simulink model "snb_bc"  (R2012b)
settings: Solver=FixedStepDiscrete  SolverMode=SingleTasking  StartTime=0.0  StopTime=10000  RelTol=1e-3
undefined symbols (not defined in the file): Down, pfb_coeff_gen_calc, Up
libraries: xbsIndex_r4 x19640, casper_library_misc x44, casper_library_delays x18, casper_library_communications x8, xps_library x3
(part 79 of 163)

== system snb_bc/pfb_fft/pfb_fir_generic/pfb_fir_taps/delay_bram ==
  addr : Inport
  din : Inport  Port=2
  we : Inport  Port=3
  en : Inport  Port=4
  bram{0..125} (126 alike) : xbsIndex_r4/Single Port RAM  depth=8192  initVector=getfield(get_param(gcb, 'UserData'), 'initVector')  distributed_mem=Block RAM  write_mode=Read Before Write  rst=off  init_reg=0  en=on  latency=8  dbl_ovrd=off  optimize=Speed  block_type=spram
  ddin : xbsIndex_r4/Delay  rst=off  infoeditControl=Selection of Reset will increase slice count due to use of real FFs and instead of SRLs  en=off  latency=0  dbl_ovrd=off  reg_retiming=on  block_type=delay
  debus_addr : Subsystem  AncestorBlock=casper_library_flow_control/bus_expand  mask(bus_expand){mode=divisions of equal size, outputNum=126, outputWidth=[13 13 13 13 13 13 13 13 13 13 13 13 13 13 13 13 13 13 13 13 13 13 13 13 13 13 13 13 13 13 13 13 13 13 13 13 13 13 13 13 13 13 13 13 13 13 13 13 13 13 13 13 13 13 13 13 13 13 13 13 13 13 13 13 13 13 13 13 13 13 13 13 13 13 13 13 13 13 13 13 13 13 13 13 13 13 13 13 13 13 13 13 13 13 13 13 13 13 13 13 13 13 13 13 13 13 13 13 13 13 13 13 13 13 13 13 13 13 13 13 13 13 13 13 13 13], outputBinaryPt=[0 0 0 0 0 0 0 0 0 0 0 0 0 0 0 0 0 0 0 0 0 0 0 0 0 0 0 0 0 0 0 0 0 0 0 0 0 0 0 0 0 0 0 0 0 0 0 0 0 0 0 0 0 0 0 0 0 0 0 0 0 0 0 0 0 0 0 0 0 0 0 0 0 0 0 0 0 0 0 0 0 0 0 0 0 0 0 0 0 0 0 0 0 0 0 0 0 0 0 0 0 0 0 0 0 0 0 0 0 0 0 0 0 0 0 0 0 0 0 0 0 0 0 0 0 0], outputArithmeticType=[0 0 0 0 0 0 0 0 0 0 0 0 0 0 0 0 0 0 0 0 0 0 0 0 0 0 0 0 0 0 0 0 0 0 0 0 0 0 0 0 0 0 0 0 0 0 0 0 0 0 0 0 0 0 0 0 0 0 0 0 0 0 0 0 0 0 0 0 0 0 0 0 0 0 0 0 0 0 0 0 0 0 0 0 0 0 0 0 0 0 0 0 0 0 0 0 0 0 0 0 0 0 0 0 0 0 0 0 0 0 0 0 0 0 0 0 0 0 0 0 0 0 0 0 0 0], show_format=on, outputToWorkspace=off, variablePrefix=, outputToModelAsWell=on}
      mask prompts: outputNum "Number of outputs:"; outputWidth "Output width:"; outputBinaryPt "Output binary point position:"; outputArithmeticType "Output arithmetic type (ufix=0, fix=1, bool=2):"; show_format "Print format string?"; outputToWorkspace "Output to workspace?"; variablePrefix "Variable name prefix:"; outputToModelAsWell "Output to model as well?"
      mask help:
      | Expands a 'bus' made using a bus_create or Xilinx
      | concat block.
      | The input will be divided into the specified number
      | of outputs with the specified arithmetic types.
      | Divisions are made from most significant bit.
      mask init: same as snb_bc/bus_expand10
      settings: AttributesFormatString=126 outputs: uf13.0,uf13.0,uf13.0,uf13.0,uf13.0,uf13.0,uf13.0,uf13.0,uf13.0,uf13.0,uf13.0,uf13.0,uf13.0,uf13.0,uf13.0,uf13.0,uf13.0,uf13.0,uf13.0,uf13.0,uf13.0,uf13.0,uf13.0,uf13.0,uf13.0,uf13.0,uf13.0,uf13.0,uf13.0,uf13.0,uf13.0,uf13.0,uf13.0,uf13.0,uf13.0,uf13.0,uf13.0,uf13.0,uf13.0,uf13.0,uf13.0,uf13.0,uf13.0,uf13.0,uf13.0,uf13.0,uf13.0,uf13.0,uf13.0,uf13.0,uf13.0,uf13.0,uf13.0,uf13.0,uf13.0,uf13.0,uf13.0,uf13.0,uf13.0,uf13.0,uf13.0,uf13.0,uf13.0,uf13.0,uf13.0,uf13.0,uf13.0,uf13.0,uf13.0,uf13.0,uf13.0,uf13.0,uf13.0,uf13.0,uf13.0,uf13.0,uf13.0,uf13.0,uf13.0,uf13.0,uf13.0,uf13.0,uf13.0,uf13.0,uf13.0,uf13.0,uf13.0,uf13.0,uf13.0,uf13.0,uf13.0,uf13.0,uf13.0,uf13.0,uf13.0,uf13.0,uf13.0,uf13.0,uf13.0,uf13.0,uf13.0,uf13.0,uf13.0,uf13.0,uf13.0,uf13.0,uf13.0,uf13.0,uf13.0,uf13.0,uf13.0,uf13.0,uf13.0,uf13.0,uf13.0,uf13.0,uf13.0,uf13.0,uf13.0,uf13.0,uf13.0,uf13.0,uf13.0,uf13.0,uf13.0,uf13.0,
      mask TypeOptions mode: divisions of equal size | divisions of arbitrary size
      mask Callback mode: bus_expand_callback();
      mask Callback outputWidth: bus_expand_callback();
      mask Callback outputToWorkspace: bus_expand_callback();
  debus_din : Subsystem  AncestorBlock=casper_library_flow_control/bus_expand  mask(bus_expand){mode=divisions of arbitrary size, outputNum=1, outputWidth=[4 4 4 4 4 4 4 4 4 4 4 4 4 4 4 4 4 4 4 4 4 4 4 4 4 4 4 4 4 4 4 4 4 4 4 4 4 4 4 4 4 4 4 4 4 4 4 4 4 4 4 4 4 4 4 4 4 4 4 4 4 4 4 4 4 4 4 4 4 4 4 4 4 4 4 4 4 4 4 4 4 4 4 4 4 4 4 4 4 4 4 4 4 4 4 4 4 4 4 4 4 4 4 4 4 4 4 4 4 4 4 4 4 4 4 4 4 4 4 4 4 4 4 4 4 4], outputBinaryPt=[0 0 0 0 0 0 0 0 0 0 0 0 0 0 0 0 0 0 0 0 0 0 0 0 0 0 0 0 0 0 0 0 0 0 0 0 0 0 0 0 0 0 0 0 0 0 0 0 0 0 0 0 0 0 0 0 0 0 0 0 0 0 0 0 0 0 0 0 0 0 0 0 0 0 0 0 0 0 0 0 0 0 0 0 0 0 0 0 0 0 0 0 0 0 0 0 0 0 0 0 0 0 0 0 0 0 0 0 0 0 0 0 0 0 0 0 0 0 0 0 0 0 0 0 0 0], outputArithmeticType=[0 0 0 0 0 0 0 0 0 0 0 0 0 0 0 0 0 0 0 0 0 0 0 0 0 0 0 0 0 0 0 0 0 0 0 0 0 0 0 0 0 0 0 0 0 0 0 0 0 0 0 0 0 0 0 0 0 0 0 0 0 0 0 0 0 0 0 0 0 0 0 0 0 0 0 0 0 0 0 0 0 0 0 0 0 0 0 0 0 0 0 0 0 0 0 0 0 0 0 0 0 0 0 0 0 0 0 0 0 0 0 0 0 0 0 0 0 0 0 0 0 0 0 0 0 0], show_format=on, outputToWorkspace=off, variablePrefix=, outputToModelAsWell=on}
      mask prompts: outputNum "Number of outputs:"; outputWidth "Output width [msb ... lsb]:"; outputBinaryPt "Output binary point position [msb ... lsb]:"; outputArithmeticType "Output arithmetic type (ufix=0, fix=1, bool=2) [msb ... lsb]:"; show_format "Print format string?"; outputToWorkspace "Output to workspace?"; variablePrefix "Variable name prefix:"; outputToModelAsWell "Output to model as well?"
      mask help:
      | Expands a 'bus' made using a bus_create or Xilinx
      | concat block.
      | The input will be divided into the specified number
      | of outputs with the specified arithmetic types.
      | Divisions are made from most significant bit.
      mask init: same as snb_bc/bus_expand10
      settings: AttributesFormatString=126 outputs: uf4.0,uf4.0,uf4.0,uf4.0,uf4.0,uf4.0,uf4.0,uf4.0,uf4.0,uf4.0,uf4.0,uf4.0,uf4.0,uf4.0,uf4.0,uf4.0,uf4.0,uf4.0,uf4.0,uf4.0,uf4.0,uf4.0,uf4.0,uf4.0,uf4.0,uf4.0,uf4.0,uf4.0,uf4.0,uf4.0,uf4.0,uf4.0,uf4.0,uf4.0,uf4.0,uf4.0,uf4.0,uf4.0,uf4.0,uf4.0,uf4.0,uf4.0,uf4.0,uf4.0,uf4.0,uf4.0,uf4.0,uf4.0,uf4.0,uf4.0,uf4.0,uf4.0,uf4.0,uf4.0,uf4.0,uf4.0,uf4.0,uf4.0,uf4.0,uf4.0,uf4.0,uf4.0,uf4.0,uf4.0,uf4.0,uf4.0,uf4.0,uf4.0,uf4.0,uf4.0,uf4.0,uf4.0,uf4.0,uf4.0,uf4.0,uf4.0,uf4.0,uf4.0,uf4.0,uf4.0,uf4.0,uf4.0,uf4.0,uf4.0,uf4.0,uf4.0,uf4.0,uf4.0,uf4.0,uf4.0,uf4.0,uf4.0,uf4.0,uf4.0,uf4.0,uf4.0,uf4.0,uf4.0,uf4.0,uf4.0,uf4.0,uf4.0,uf4.0,uf4.0,uf4.0,uf4.0,uf4.0,uf4.0,uf4.0,uf4.0,uf4.0,uf4.0,uf4.0,uf4.0,uf4.0,uf4.0,uf4.0,uf4.0,uf4.0,uf4.0,uf4.0,uf4.0,uf4.0,uf4.0,uf4.0,uf4.0,
      mask TypeOptions mode: divisions of equal size | divisions of arbitrary size
      mask Callback mode: bus_expand_callback();
      mask Callback outputWidth: bus_expand_callback();
      mask Callback outputToWorkspace: bus_expand_callback();
  debus_en : Subsystem  AncestorBlock=casper_library_flow_control/bus_expand  mask(bus_expand){mode=divisions of equal size, outputNum=126, outputWidth=[1 1 1 1 1 1 1 1 1 1 1 1 1 1 1 1 1 1 1 1 1 1 1 1 1 1 1 1 1 1 1 1 1 1 1 1 1 1 1 1 1 1 1 1 1 1 1 1 1 1 1 1 1 1 1 1 1 1 1 1 1 1 1 1 1 1 1 1 1 1 1 1 1 1 1 1 1 1 1 1 1 1 1 1 1 1 1 1 1 1 1 1 1 1 1 1 1 1 1 1 1 1 1 1 1 1 1 1 1 1 1 1 1 1 1 1 1 1 1 1 1 1 1 1 1 1], outputBinaryPt=[0 0 0 0 0 0 0 0 0 0 0 0 0 0 0 0 0 0 0 0 0 0 0 0 0 0 0 0 0 0 0 0 0 0 0 0 0 0 0 0 0 0 0 0 0 0 0 0 0 0 0 0 0 0 0 0 0 0 0 0 0 0 0 0 0 0 0 0 0 0 0 0 0 0 0 0 0 0 0 0 0 0 0 0 0 0 0 0 0 0 0 0 0 0 0 0 0 0 0 0 0 0 0 0 0 0 0 0 0 0 0 0 0 0 0 0 0 0 0 0 0 0 0 0 0 0], outputArithmeticType=[2 2 2 2 2 2 2 2 2 2 2 2 2 2 2 2 2 2 2 2 2 2 2 2 2 2 2 2 2 2 2 2 2 2 2 2 2 2 2 2 2 2 2 2 2 2 2 2 2 2 2 2 2 2 2 2 2 2 2 2 2 2 2 2 2 2 2 2 2 2 2 2 2 2 2 2 2 2 2 2 2 2 2 2 2 2 2 2 2 2 2 2 2 2 2 2 2 2 2 2 2 2 2 2 2 2 2 2 2 2 2 2 2 2 2 2 2 2 2 2 2 2 2 2 2 2], show_format=on, outputToWorkspace=off, variablePrefix=, outputToModelAsWell=on}
      mask prompts: outputNum "Number of outputs:"; outputWidth "Output width:"; outputBinaryPt "Output binary point position:"; outputArithmeticType "Output arithmetic type (ufix=0, fix=1, bool=2):"; show_format "Print format string?"; outputToWorkspace "Output to workspace?"; variablePrefix "Variable name prefix:"; outputToModelAsWell "Output to model as well?"
      mask help:
      | Expands a 'bus' made using a bus_create or Xilinx
      | concat block.
      | The input will be divided into the specified number
      | of outputs with the specified arithmetic types.
      | Divisions are made from most significant bit.
      mask init: same as snb_bc/bus_expand10
      settings: AttributesFormatString=126 outputs: b,b,b,b,b,b,b,b,b,b,b,b,b,b,b,b,b,b,b,b,b,b,b,b,b,b,b,b,b,b,b,b,b,b,b,b,b,b,b,b,b,b,b,b,b,b,b,b,b,b,b,b,b,b,b,b,b,b,b,b,b,b,b,b,b,b,b,b,b,b,b,b,b,b,b,b,b,b,b,b,b,b,b,b,b,b,b,b,b,b,b,b,b,b,b,b,b,b,b,b,b,b,b,b,b,b,b,b,b,b,b,b,b,b,b,b,b,b,b,b,b,b,b,b,b,b,
      mask TypeOptions mode: divisions of equal size | divisions of arbitrary size
      mask Callback mode: bus_expand_callback();
      mask Callback outputWidth: bus_expand_callback();
      mask Callback outputToWorkspace: bus_expand_callback();
  debus_we : Subsystem  AncestorBlock=casper_library_flow_control/bus_expand  mask(bus_expand){mode=divisions of equal size, outputNum=126, outputWidth=[1 1 1 1 1 1 1 1 1 1 1 1 1 1 1 1 1 1 1 1 1 1 1 1 1 1 1 1 1 1 1 1 1 1 1 1 1 1 1 1 1 1 1 1 1 1 1 1 1 1 1 1 1 1 1 1 1 1 1 1 1 1 1 1 1 1 1 1 1 1 1 1 1 1 1 1 1 1 1 1 1 1 1 1 1 1 1 1 1 1 1 1 1 1 1 1 1 1 1 1 1 1 1 1 1 1 1 1 1 1 1 1 1 1 1 1 1 1 1 1 1 1 1 1 1 1], outputBinaryPt=[0 0 0 0 0 0 0 0 0 0 0 0 0 0 0 0 0 0 0 0 0 0 0 0 0 0 0 0 0 0 0 0 0 0 0 0 0 0 0 0 0 0 0 0 0 0 0 0 0 0 0 0 0 0 0 0 0 0 0 0 0 0 0 0 0 0 0 0 0 0 0 0 0 0 0 0 0 0 0 0 0 0 0 0 0 0 0 0 0 0 0 0 0 0 0 0 0 0 0 0 0 0 0 0 0 0 0 0 0 0 0 0 0 0 0 0 0 0 0 0 0 0 0 0 0 0], outputArithmeticType=[2 2 2 2 2 2 2 2 2 2 2 2 2 2 2 2 2 2 2 2 2 2 2 2 2 2 2 2 2 2 2 2 2 2 2 2 2 2 2 2 2 2 2 2 2 2 2 2 2 2 2 2 2 2 2 2 2 2 2 2 2 2 2 2 2 2 2 2 2 2 2 2 2 2 2 2 2 2 2 2 2 2 2 2 2 2 2 2 2 2 2 2 2 2 2 2 2 2 2 2 2 2 2 2 2 2 2 2 2 2 2 2 2 2 2 2 2 2 2 2 2 2 2 2 2 2], show_format=on, outputToWorkspace=off, variablePrefix=, outputToModelAsWell=on}
      mask prompts: outputNum "Number of outputs:"; outputWidth "Output width:"; outputBinaryPt "Output binary point position:"; outputArithmeticType "Output arithmetic type (ufix=0, fix=1, bool=2):"; show_format "Print format string?"; outputToWorkspace "Output to workspace?"; variablePrefix "Variable name prefix:"; outputToModelAsWell "Output to model as well?"
      mask help:
      | Expands a 'bus' made using a bus_create or Xilinx
      | concat block.
      | The input will be divided into the specified number
      | of outputs with the specified arithmetic types.
      | Divisions are made from most significant bit.
      mask init: same as snb_bc/bus_expand10
      settings: AttributesFormatString=126 outputs: b,b,b,b,b,b,b,b,b,b,b,b,b,b,b,b,b,b,b,b,b,b,b,b,b,b,b,b,b,b,b,b,b,b,b,b,b,b,b,b,b,b,b,b,b,b,b,b,b,b,b,b,b,b,b,b,b,b,b,b,b,b,b,b,b,b,b,b,b,b,b,b,b,b,b,b,b,b,b,b,b,b,b,b,b,b,b,b,b,b,b,b,b,b,b,b,b,b,b,b,b,b,b,b,b,b,b,b,b,b,b,b,b,b,b,b,b,b,b,b,b,b,b,b,b,b,
      mask TypeOptions mode: divisions of equal size | divisions of arbitrary size
      mask Callback mode: bus_expand_callback();
      mask Callback outputWidth: bus_expand_callback();
      mask Callback outputToWorkspace: bus_expand_callback();
  den : xbsIndex_r4/Delay  rst=off  infoeditControl=Selection of Reset will increase slice count due to use of real FFs and instead of SRLs  en=off  latency=8  dbl_ovrd=off  reg_retiming=on  block_type=delay
  din_bussify : Subsystem  AncestorBlock=casper_library_flow_control/bus_create  mask(bus_create){inputNum=126}
      mask prompts: inputNum "Number of inputs:"
      mask init:
      | bus_create_init(gcb,...
      |     'inputNum', inputNum);
  rep_addr : Subsystem  AncestorBlock=casper_library_bus/bus_replicate  mask(bus_replicate){replication=126, latency=9, misc=off, implementation=core}
      mask prompts: replication "replication factor"; misc "misc support"; implementation "delay implementation"
      mask help: Output bus formed by replicating input bus a number of times
      mask init:
      | bus_replicate_init(gcb, ...
      |     'replication', replication, ...
      |     'latency', latency, ...
      |     'implementation', implementation, ...
      |     'misc', misc);
      mask TypeOptions implementation: core | behavioral
  rep_en : Subsystem  AncestorBlock=casper_library_bus/bus_replicate  mask(bus_replicate){replication=126, latency=9, misc=off, implementation=core}
      mask prompts: replication "replication factor"; misc "misc support"; implementation "delay implementation"
      mask help: Output bus formed by replicating input bus a number of times
      mask init:
      | bus_replicate_init(gcb, ...
      |     'replication', replication, ...
      |     'latency', latency, ...
      |     'implementation', implementation, ...
      |     'misc', misc);
      mask TypeOptions implementation: core | behavioral
  rep_we : Subsystem  AncestorBlock=casper_library_bus/bus_replicate  mask(bus_replicate){replication=126, latency=0, misc=off, implementation=behavioral}
      mask prompts: replication "replication factor"; misc "misc support"; implementation "delay implementation"
      mask help: Output bus formed by replicating input bus a number of times
      mask init:
      | bus_replicate_init(gcb, ...
      |     'replication', replication, ...
      |     'latency', latency, ...
      |     'implementation', implementation, ...
      |     'misc', misc);
      mask TypeOptions implementation: core | behavioral
  dout : Outport
  dvalid : Outport  Port=2
  wires:
  addr/1 -> rep_addr/1(in)
  din/1 -> ddin/1
  we/1 -> rep_we/1(in)
  en/1 -> rep_en/1(in)
  rep_addr/1(out) -> debus_addr/1(bus_in)
  ddin/1 -> debus_din/1(bus_in)
  rep_we/1(out) -> debus_we/1(bus_in)
  rep_en/1(out) -> debus_en/1(bus_in)
  debus_addr/1(msb_out126) -> bram0/1
  debus_din/1(msb_out126) -> bram0/2
  debus_we/1(msb_out126) -> bram0/3
  debus_en/1(msb_out126) -> bram0/4
  debus_addr/2(out125) -> bram1/1
  debus_din/2(out125) -> bram1/2
  debus_we/2(out125) -> bram1/3
  debus_en/2(out125) -> bram1/4
  debus_addr/3(out124) -> bram2/1
  debus_din/3(out124) -> bram2/2
  debus_we/3(out124) -> bram2/3
  debus_en/3(out124) -> bram2/4
  debus_addr/4(out123) -> bram3/1
  debus_din/4(out123) -> bram3/2
  debus_we/4(out123) -> bram3/3
  debus_en/4(out123) -> bram3/4
  debus_addr/5(out122) -> bram4/1
  debus_din/5(out122) -> bram4/2
  debus_we/5(out122) -> bram4/3
  debus_en/5(out122) -> bram4/4
  debus_addr/6(out121) -> bram5/1
  debus_din/6(out121) -> bram5/2
  debus_we/6(out121) -> bram5/3
  debus_en/6(out121) -> bram5/4
  debus_addr/7(out120) -> bram6/1
  debus_din/7(out120) -> bram6/2
  debus_we/7(out120) -> bram6/3
  debus_en/7(out120) -> bram6/4
  debus_addr/8(out119) -> bram7/1
  debus_din/8(out119) -> bram7/2
  debus_we/8(out119) -> bram7/3
  debus_en/8(out119) -> bram7/4
  debus_addr/9(out118) -> bram8/1
  debus_din/9(out118) -> bram8/2
  debus_we/9(out118) -> bram8/3
  debus_en/9(out118) -> bram8/4
  debus_addr/10(out117) -> bram9/1
  debus_din/10(out117) -> bram9/2
  debus_we/10(out117) -> bram9/3
  debus_en/10(out117) -> bram9/4
  debus_addr/11(out116) -> bram10/1
  debus_din/11(out116) -> bram10/2
  debus_we/11(out116) -> bram10/3
  debus_en/11(out116) -> bram10/4
  debus_addr/12(out115) -> bram11/1
  debus_din/12(out115) -> bram11/2
  debus_we/12(out115) -> bram11/3
  debus_en/12(out115) -> bram11/4
  debus_addr/13(out114) -> bram12/1
  debus_din/13(out114) -> bram12/2
  debus_we/13(out114) -> bram12/3
  debus_en/13(out114) -> bram12/4
  debus_addr/14(out113) -> bram13/1
  debus_din/14(out113) -> bram13/2
  debus_we/14(out113) -> bram13/3
  debus_en/14(out113) -> bram13/4
  debus_addr/15(out112) -> bram14/1
  debus_din/15(out112) -> bram14/2
  debus_we/15(out112) -> bram14/3
  debus_en/15(out112) -> bram14/4
  debus_addr/16(out111) -> bram15/1
  debus_din/16(out111) -> bram15/2
  debus_we/16(out111) -> bram15/3
  debus_en/16(out111) -> bram15/4
  debus_addr/17(out110) -> bram16/1
  debus_din/17(out110) -> bram16/2
  debus_we/17(out110) -> bram16/3
  debus_en/17(out110) -> bram16/4
  debus_addr/18(out109) -> bram17/1
  debus_din/18(out109) -> bram17/2
  debus_we/18(out109) -> bram17/3
  debus_en/18(out109) -> bram17/4
  debus_addr/19(out108) -> bram18/1
  debus_din/19(out108) -> bram18/2
  debus_we/19(out108) -> bram18/3
  debus_en/19(out108) -> bram18/4
  debus_addr/20(out107) -> bram19/1
  debus_din/20(out107) -> bram19/2
  debus_we/20(out107) -> bram19/3
  debus_en/20(out107) -> bram19/4
  debus_addr/21(out106) -> bram20/1
  debus_din/21(out106) -> bram20/2
  debus_we/21(out106) -> bram20/3
  debus_en/21(out106) -> bram20/4
  debus_addr/22(out105) -> bram21/1
  debus_din/22(out105) -> bram21/2
  debus_we/22(out105) -> bram21/3
  debus_en/22(out105) -> bram21/4
  debus_addr/23(out104) -> bram22/1
  debus_din/23(out104) -> bram22/2
  debus_we/23(out104) -> bram22/3
  debus_en/23(out104) -> bram22/4
  debus_addr/24(out103) -> bram23/1
  debus_din/24(out103) -> bram23/2
  debus_we/24(out103) -> bram23/3
  debus_en/24(out103) -> bram23/4
  debus_addr/25(out102) -> bram24/1
  debus_din/25(out102) -> bram24/2
  debus_we/25(out102) -> bram24/3
  debus_en/25(out102) -> bram24/4
  debus_addr/26(out101) -> bram25/1
  debus_din/26(out101) -> bram25/2
  debus_we/26(out101) -> bram25/3
  debus_en/26(out101) -> bram25/4
  debus_addr/27(out100) -> bram26/1
  debus_din/27(out100) -> bram26/2
  debus_we/27(out100) -> bram26/3
  debus_en/27(out100) -> bram26/4
  debus_addr/28(out99) -> bram27/1
  debus_din/28(out99) -> bram27/2
  debus_we/28(out99) -> bram27/3
  debus_en/28(out99) -> bram27/4
  debus_addr/29(out98) -> bram28/1
  debus_din/29(out98) -> bram28/2
  debus_we/29(out98) -> bram28/3
  debus_en/29(out98) -> bram28/4
  debus_addr/30(out97) -> bram29/1
  debus_din/30(out97) -> bram29/2
  debus_we/30(out97) -> bram29/3
  debus_en/30(out97) -> bram29/4
  debus_addr/31(out96) -> bram30/1
  debus_din/31(out96) -> bram30/2
  debus_we/31(out96) -> bram30/3
  debus_en/31(out96) -> bram30/4
  debus_addr/32(out95) -> bram31/1
  debus_din/32(out95) -> bram31/2
  debus_we/32(out95) -> bram31/3
  debus_en/32(out95) -> bram31/4
  debus_addr/33(out94) -> bram32/1
  debus_din/33(out94) -> bram32/2
  debus_we/33(out94) -> bram32/3
  debus_en/33(out94) -> bram32/4
  debus_addr/34(out93) -> bram33/1
  debus_din/34(out93) -> bram33/2
  debus_we/34(out93) -> bram33/3
  debus_en/34(out93) -> bram33/4
  debus_addr/35(out92) -> bram34/1
  debus_din/35(out92) -> bram34/2
  debus_we/35(out92) -> bram34/3
  debus_en/35(out92) -> bram34/4
  debus_addr/36(out91) -> bram35/1
  debus_din/36(out91) -> bram35/2
  debus_we/36(out91) -> bram35/3
  debus_en/36(out91) -> bram35/4
  debus_addr/37(out90) -> bram36/1
  debus_din/37(out90) -> bram36/2
  debus_we/37(out90) -> bram36/3
  debus_en/37(out90) -> bram36/4
  debus_addr/38(out89) -> bram37/1
  debus_din/38(out89) -> bram37/2
  debus_we/38(out89) -> bram37/3
  debus_en/38(out89) -> bram37/4
  debus_addr/39(out88) -> bram38/1
  debus_din/39(out88) -> bram38/2
  debus_we/39(out88) -> bram38/3
  debus_en/39(out88) -> bram38/4
  debus_addr/40(out87) -> bram39/1
  debus_din/40(out87) -> bram39/2
  debus_we/40(out87) -> bram39/3
  debus_en/40(out87) -> bram39/4
  debus_addr/41(out86) -> bram40/1
  debus_din/41(out86) -> bram40/2
  debus_we/41(out86) -> bram40/3
  debus_en/41(out86) -> bram40/4
  debus_addr/42(out85) -> bram41/1
  debus_din/42(out85) -> bram41/2
  debus_we/42(out85) -> bram41/3
  debus_en/42(out85) -> bram41/4
  debus_addr/43(out84) -> bram42/1
  debus_din/43(out84) -> bram42/2
  debus_we/43(out84) -> bram42/3
  debus_en/43(out84) -> bram42/4
  debus_addr/44(out83) -> bram43/1
  debus_din/44(out83) -> bram43/2
  debus_we/44(out83) -> bram43/3
  debus_en/44(out83) -> bram43/4
  debus_addr/45(out82) -> bram44/1
  debus_din/45(out82) -> bram44/2
  debus_we/45(out82) -> bram44/3
  debus_en/45(out82) -> bram44/4
  debus_addr/46(out81) -> bram45/1
  debus_din/46(out81) -> bram45/2
  debus_we/46(out81) -> bram45/3
  debus_en/46(out81) -> bram45/4
  debus_addr/47(out80) -> bram46/1
  debus_din/47(out80) -> bram46/2
  debus_we/47(out80) -> bram46/3
  debus_en/47(out80) -> bram46/4
  debus_addr/48(out79) -> bram47/1
  debus_din/48(out79) -> bram47/2
  debus_we/48(out79) -> bram47/3
  debus_en/48(out79) -> bram47/4
  debus_addr/49(out78) -> bram48/1
  debus_din/49(out78) -> bram48/2
  debus_we/49(out78) -> bram48/3
  debus_en/49(out78) -> bram48/4
  debus_addr/50(out77) -> bram49/1
  debus_din/50(out77) -> bram49/2
  debus_we/50(out77) -> bram49/3
  debus_en/50(out77) -> bram49/4
  debus_addr/51(out76) -> bram50/1
  debus_din/51(out76) -> bram50/2
  debus_we/51(out76) -> bram50/3
  debus_en/51(out76) -> bram50/4
  debus_addr/52(out75) -> bram51/1
  debus_din/52(out75) -> bram51/2
  debus_we/52(out75) -> bram51/3
  debus_en/52(out75) -> bram51/4
  debus_addr/53(out74) -> bram52/1
  debus_din/53(out74) -> bram52/2
  debus_we/53(out74) -> bram52/3
  debus_en/53(out74) -> bram52/4
  debus_addr/54(out73) -> bram53/1
  debus_din/54(out73) -> bram53/2
  debus_we/54(out73) -> bram53/3
  debus_en/54(out73) -> bram53/4
  debus_addr/55(out72) -> bram54/1
  debus_din/55(out72) -> bram54/2
  debus_we/55(out72) -> bram54/3
  debus_en/55(out72) -> bram54/4
  debus_addr/56(out71) -> bram55/1
  debus_din/56(out71) -> bram55/2
  debus_we/56(out71) -> bram55/3
  debus_en/56(out71) -> bram55/4
  debus_addr/57(out70) -> bram56/1
  debus_din/57(out70) -> bram56/2
  debus_we/57(out70) -> bram56/3
  debus_en/57(out70) -> bram56/4
  debus_addr/58(out69) -> bram57/1
  debus_din/58(out69) -> bram57/2
  debus_we/58(out69) -> bram57/3
  debus_en/58(out69) -> bram57/4
  debus_addr/59(out68) -> bram58/1
  debus_din/59(out68) -> bram58/2
  debus_we/59(out68) -> bram58/3
  debus_en/59(out68) -> bram58/4
  debus_addr/60(out67) -> bram59/1
  debus_din/60(out67) -> bram59/2
  debus_we/60(out67) -> bram59/3
  debus_en/60(out67) -> bram59/4
  debus_addr/61(out66) -> bram60/1
  debus_din/61(out66) -> bram60/2
  debus_we/61(out66) -> bram60/3
  debus_en/61(out66) -> bram60/4
  debus_addr/62(out65) -> bram61/1
  debus_din/62(out65) -> bram61/2
  debus_we/62(out65) -> bram61/3
  debus_en/62(out65) -> bram61/4
  debus_addr/63(out64) -> bram62/1
  debus_din/63(out64) -> bram62/2
  debus_we/63(out64) -> bram62/3
  debus_en/63(out64) -> bram62/4
  debus_addr/64(out63) -> bram63/1
  debus_din/64(out63) -> bram63/2
  debus_we/64(out63) -> bram63/3
  debus_en/64(out63) -> bram63/4
  debus_addr/65(out62) -> bram64/1
  debus_din/65(out62) -> bram64/2
  debus_we/65(out62) -> bram64/3
  debus_en/65(out62) -> bram64/4
  debus_addr/66(out61) -> bram65/1
  debus_din/66(out61) -> bram65/2
  debus_we/66(out61) -> bram65/3
  debus_en/66(out61) -> bram65/4
  debus_addr/67(out60) -> bram66/1
  debus_din/67(out60) -> bram66/2
  debus_we/67(out60) -> bram66/3
  debus_en/67(out60) -> bram66/4
  debus_addr/68(out59) -> bram67/1
  debus_din/68(out59) -> bram67/2
  debus_we/68(out59) -> bram67/3
  debus_en/68(out59) -> bram67/4
  debus_addr/69(out58) -> bram68/1
  debus_din/69(out58) -> bram68/2
  debus_we/69(out58) -> bram68/3
  debus_en/69(out58) -> bram68/4
  debus_addr/70(out57) -> bram69/1
  debus_din/70(out57) -> bram69/2
  debus_we/70(out57) -> bram69/3
  debus_en/70(out57) -> bram69/4
  debus_addr/71(out56) -> bram70/1
  debus_din/71(out56) -> bram70/2
  debus_we/71(out56) -> bram70/3
  debus_en/71(out56) -> bram70/4
  debus_addr/72(out55) -> bram71/1
  debus_din/72(out55) -> bram71/2
  debus_we/72(out55) -> bram71/3
  debus_en/72(out55) -> bram71/4
  debus_addr/73(out54) -> bram72/1
  debus_din/73(out54) -> bram72/2
  debus_we/73(out54) -> bram72/3
  debus_en/73(out54) -> bram72/4
  debus_addr/74(out53) -> bram73/1
  debus_din/74(out53) -> bram73/2
  debus_we/74(out53) -> bram73/3
  debus_en/74(out53) -> bram73/4
  debus_addr/75(out52) -> bram74/1
  debus_din/75(out52) -> bram74/2
  debus_we/75(out52) -> bram74/3
  debus_en/75(out52) -> bram74/4
  debus_addr/76(out51) -> bram75/1
  debus_din/76(out51) -> bram75/2
  debus_we/76(out51) -> bram75/3
  debus_en/76(out51) -> bram75/4
  debus_addr/77(out50) -> bram76/1
  debus_din/77(out50) -> bram76/2
  debus_we/77(out50) -> bram76/3
  debus_en/77(out50) -> bram76/4
  debus_addr/78(out49) -> bram77/1
  debus_din/78(out49) -> bram77/2
  debus_we/78(out49) -> bram77/3
  debus_en/78(out49) -> bram77/4
  debus_addr/79(out48) -> bram78/1
  debus_din/79(out48) -> bram78/2
  debus_we/79(out48) -> bram78/3
  debus_en/79(out48) -> bram78/4
  debus_addr/80(out47) -> bram79/1
  debus_din/80(out47) -> bram79/2
  debus_we/80(out47) -> bram79/3
  debus_en/80(out47) -> bram79/4
  debus_addr/81(out46) -> bram80/1
  debus_din/81(out46) -> bram80/2
  debus_we/81(out46) -> bram80/3
  debus_en/81(out46) -> bram80/4
  debus_addr/82(out45) -> bram81/1
  debus_din/82(out45) -> bram81/2
  debus_we/82(out45) -> bram81/3
  debus_en/82(out45) -> bram81/4
  debus_addr/83(out44) -> bram82/1
  debus_din/83(out44) -> bram82/2
  debus_we/83(out44) -> bram82/3
  debus_en/83(out44) -> bram82/4
  debus_addr/84(out43) -> bram83/1
  debus_din/84(out43) -> bram83/2
  debus_we/84(out43) -> bram83/3
  debus_en/84(out43) -> bram83/4
  debus_addr/85(out42) -> bram84/1
  debus_din/85(out42) -> bram84/2
  debus_we/85(out42) -> bram84/3
  debus_en/85(out42) -> bram84/4
  debus_addr/86(out41) -> bram85/1
  debus_din/86(out41) -> bram85/2
  debus_we/86(out41) -> bram85/3
  debus_en/86(out41) -> bram85/4
  debus_addr/87(out40) -> bram86/1
  debus_din/87(out40) -> bram86/2
  debus_we/87(out40) -> bram86/3
  debus_en/87(out40) -> bram86/4
  debus_addr/88(out39) -> bram87/1
  debus_din/88(out39) -> bram87/2
  debus_we/88(out39) -> bram87/3
  debus_en/88(out39) -> bram87/4
  debus_addr/89(out38) -> bram88/1
  debus_din/89(out38) -> bram88/2
  debus_we/89(out38) -> bram88/3
  debus_en/89(out38) -> bram88/4
  debus_addr/90(out37) -> bram89/1
  debus_din/90(out37) -> bram89/2
  debus_we/90(out37) -> bram89/3
  debus_en/90(out37) -> bram89/4
  debus_addr/91(out36) -> bram90/1
  debus_din/91(out36) -> bram90/2
  debus_we/91(out36) -> bram90/3
  debus_en/91(out36) -> bram90/4
  debus_addr/92(out35) -> bram91/1
  debus_din/92(out35) -> bram91/2
  debus_we/92(out35) -> bram91/3
  debus_en/92(out35) -> bram91/4
  debus_addr/93(out34) -> bram92/1
  debus_din/93(out34) -> bram92/2
  debus_we/93(out34) -> bram92/3
  debus_en/93(out34) -> bram92/4
  debus_addr/94(out33) -> bram93/1
  debus_din/94(out33) -> bram93/2
  debus_we/94(out33) -> bram93/3
  debus_en/94(out33) -> bram93/4
  debus_addr/95(out32) -> bram94/1
  debus_din/95(out32) -> bram94/2
  debus_we/95(out32) -> bram94/3
  debus_en/95(out32) -> bram94/4
  debus_addr/96(out31) -> bram95/1
  debus_din/96(out31) -> bram95/2
  debus_we/96(out31) -> bram95/3
  debus_en/96(out31) -> bram95/4
  debus_addr/97(out30) -> bram96/1
  debus_din/97(out30) -> bram96/2
  debus_we/97(out30) -> bram96/3
  debus_en/97(out30) -> bram96/4
  debus_addr/98(out29) -> bram97/1
  debus_din/98(out29) -> bram97/2
  debus_we/98(out29) -> bram97/3
  debus_en/98(out29) -> bram97/4
  debus_addr/99(out28) -> bram98/1
  debus_din/99(out28) -> bram98/2
  debus_we/99(out28) -> bram98/3
  debus_en/99(out28) -> bram98/4
  debus_addr/100(out27) -> bram99/1
  debus_din/100(out27) -> bram99/2
  debus_we/100(out27) -> bram99/3
  debus_en/100(out27) -> bram99/4
  debus_addr/101(out26) -> bram100/1
  debus_din/101(out26) -> bram100/2
  debus_we/101(out26) -> bram100/3
  debus_en/101(out26) -> bram100/4
  debus_addr/102(out25) -> bram101/1
  debus_din/102(out25) -> bram101/2
  debus_we/102(out25) -> bram101/3
  debus_en/102(out25) -> bram101/4
  debus_addr/103(out24) -> bram102/1
  debus_din/103(out24) -> bram102/2
  debus_we/103(out24) -> bram102/3
  debus_en/103(out24) -> bram102/4
  debus_addr/104(out23) -> bram103/1
  debus_din/104(out23) -> bram103/2
  debus_we/104(out23) -> bram103/3
  debus_en/104(out23) -> bram103/4
  debus_addr/105(out22) -> bram104/1
  debus_din/105(out22) -> bram104/2
  debus_we/105(out22) -> bram104/3
  debus_en/105(out22) -> bram104/4
  debus_addr/106(out21) -> bram105/1
  debus_din/106(out21) -> bram105/2
  debus_we/106(out21) -> bram105/3
  debus_en/106(out21) -> bram105/4
  debus_addr/107(out20) -> bram106/1
  debus_din/107(out20) -> bram106/2
  debus_we/107(out20) -> bram106/3
  debus_en/107(out20) -> bram106/4
  debus_addr/108(out19) -> bram107/1
  debus_din/108(out19) -> bram107/2
  debus_we/108(out19) -> bram107/3
  debus_en/108(out19) -> bram107/4
  debus_addr/109(out18) -> bram108/1
  debus_din/109(out18) -> bram108/2
  debus_we/109(out18) -> bram108/3
  debus_en/109(out18) -> bram108/4
  debus_addr/110(out17) -> bram109/1
  debus_din/110(out17) -> bram109/2
  debus_we/110(out17) -> bram109/3
  debus_en/110(out17) -> bram109/4
  debus_addr/111(out16) -> bram110/1
  debus_din/111(out16) -> bram110/2
  debus_we/111(out16) -> bram110/3
  debus_en/111(out16) -> bram110/4
  debus_addr/112(out15) -> bram111/1
  debus_din/112(out15) -> bram111/2
  debus_we/112(out15) -> bram111/3
  debus_en/112(out15) -> bram111/4
  debus_addr/113(out14) -> bram112/1
  debus_din/113(out14) -> bram112/2
  debus_we/113(out14) -> bram112/3
  debus_en/113(out14) -> bram112/4
  debus_addr/114(out13) -> bram113/1
  debus_din/114(out13) -> bram113/2
  debus_we/114(out13) -> bram113/3
  debus_en/114(out13) -> bram113/4
  debus_addr/115(out12) -> bram114/1
  debus_din/115(out12) -> bram114/2
  debus_we/115(out12) -> bram114/3
  debus_en/115(out12) -> bram114/4
  debus_addr/116(out11) -> bram115/1
  debus_din/116(out11) -> bram115/2
  debus_we/116(out11) -> bram115/3
  debus_en/116(out11) -> bram115/4
  debus_addr/117(out10) -> bram116/1
  debus_din/117(out10) -> bram116/2
  debus_we/117(out10) -> bram116/3
  debus_en/117(out10) -> bram116/4
  debus_addr/118(out9) -> bram117/1
  debus_din/118(out9) -> bram117/2
  debus_we/118(out9) -> bram117/3
  debus_en/118(out9) -> bram117/4
  debus_addr/119(out8) -> bram118/1
  debus_din/119(out8) -> bram118/2
  debus_we/119(out8) -> bram118/3
  debus_en/119(out8) -> bram118/4
  debus_addr/120(out7) -> bram119/1
  debus_din/120(out7) -> bram119/2
  debus_we/120(out7) -> bram119/3
  debus_en/120(out7) -> bram119/4
  debus_addr/121(out6) -> bram120/1
  debus_din/121(out6) -> bram120/2
  debus_we/121(out6) -> bram120/3
  debus_en/121(out6) -> bram120/4
  debus_addr/122(out5) -> bram121/1
  debus_din/122(out5) -> bram121/2
  debus_we/122(out5) -> bram121/3
  debus_en/122(out5) -> bram121/4
  debus_addr/123(out4) -> bram122/1
  debus_din/123(out4) -> bram122/2
  debus_we/123(out4) -> bram122/3
  debus_en/123(out4) -> bram122/4
  debus_addr/124(out3) -> bram123/1
  debus_din/124(out3) -> bram123/2
  debus_we/124(out3) -> bram123/3
  debus_en/124(out3) -> bram123/4
  debus_addr/125(out2) -> bram124/1
  debus_din/125(out2) -> bram124/2
  debus_we/125(out2) -> bram124/3
  debus_en/125(out2) -> bram124/4
  debus_addr/126(lsb_out1) -> bram125/1
  debus_din/126(lsb_out1) -> bram125/2
  debus_we/126(lsb_out1) -> bram125/3
  debus_en/126(lsb_out1) -> bram125/4, den/1
  bram0/1 -> din_bussify/1(in1)
  bram1/1 -> din_bussify/2(in2)
  bram2/1 -> din_bussify/3(in3)
  bram3/1 -> din_bussify/4(in4)
  bram4/1 -> din_bussify/5(in5)
  bram5/1 -> din_bussify/6(in6)
  bram6/1 -> din_bussify/7(in7)
  bram7/1 -> din_bussify/8(in8)
  bram8/1 -> din_bussify/9(in9)
  bram9/1 -> din_bussify/10(in10)
  bram10/1 -> din_bussify/11(in11)
  bram11/1 -> din_bussify/12(in12)
  bram12/1 -> din_bussify/13(in13)
  bram13/1 -> din_bussify/14(in14)
  bram14/1 -> din_bussify/15(in15)
  bram15/1 -> din_bussify/16(in16)
  bram16/1 -> din_bussify/17(in17)
  bram17/1 -> din_bussify/18(in18)
  bram18/1 -> din_bussify/19(in19)
  bram19/1 -> din_bussify/20(in20)
  bram20/1 -> din_bussify/21(in21)
  bram21/1 -> din_bussify/22(in22)
  bram22/1 -> din_bussify/23(in23)
  bram23/1 -> din_bussify/24(in24)
  bram24/1 -> din_bussify/25(in25)
  bram25/1 -> din_bussify/26(in26)
  bram26/1 -> din_bussify/27(in27)
  bram27/1 -> din_bussify/28(in28)
  bram28/1 -> din_bussify/29(in29)
  bram29/1 -> din_bussify/30(in30)
  bram30/1 -> din_bussify/31(in31)
  bram31/1 -> din_bussify/32(in32)
  bram32/1 -> din_bussify/33(in33)
  bram33/1 -> din_bussify/34(in34)
  bram34/1 -> din_bussify/35(in35)
  bram35/1 -> din_bussify/36(in36)
  bram36/1 -> din_bussify/37(in37)
  bram37/1 -> din_bussify/38(in38)
  bram38/1 -> din_bussify/39(in39)
  bram39/1 -> din_bussify/40(in40)
  bram40/1 -> din_bussify/41(in41)
  bram41/1 -> din_bussify/42(in42)
  bram42/1 -> din_bussify/43(in43)
  bram43/1 -> din_bussify/44(in44)
  bram44/1 -> din_bussify/45(in45)
  bram45/1 -> din_bussify/46(in46)
  bram46/1 -> din_bussify/47(in47)
  bram47/1 -> din_bussify/48(in48)
  bram48/1 -> din_bussify/49(in49)
  bram49/1 -> din_bussify/50(in50)
  bram50/1 -> din_bussify/51(in51)
  bram51/1 -> din_bussify/52(in52)
  bram52/1 -> din_bussify/53(in53)
  bram53/1 -> din_bussify/54(in54)
  bram54/1 -> din_bussify/55(in55)
  bram55/1 -> din_bussify/56(in56)
  bram56/1 -> din_bussify/57(in57)
  bram57/1 -> din_bussify/58(in58)
  bram58/1 -> din_bussify/59(in59)
  bram59/1 -> din_bussify/60(in60)
  bram60/1 -> din_bussify/61(in61)
  bram61/1 -> din_bussify/62(in62)
  bram62/1 -> din_bussify/63(in63)
  bram63/1 -> din_bussify/64(in64)
  bram64/1 -> din_bussify/65(in65)
  bram65/1 -> din_bussify/66(in66)
  bram66/1 -> din_bussify/67(in67)
  bram67/1 -> din_bussify/68(in68)
  bram68/1 -> din_bussify/69(in69)
  bram69/1 -> din_bussify/70(in70)
  bram70/1 -> din_bussify/71(in71)
  bram71/1 -> din_bussify/72(in72)
  bram72/1 -> din_bussify/73(in73)
  bram73/1 -> din_bussify/74(in74)
  bram74/1 -> din_bussify/75(in75)
  bram75/1 -> din_bussify/76(in76)
  bram76/1 -> din_bussify/77(in77)
  bram77/1 -> din_bussify/78(in78)
  bram78/1 -> din_bussify/79(in79)
  bram79/1 -> din_bussify/80(in80)
  bram80/1 -> din_bussify/81(in81)
  bram81/1 -> din_bussify/82(in82)
  bram82/1 -> din_bussify/83(in83)
  bram83/1 -> din_bussify/84(in84)
  bram84/1 -> din_bussify/85(in85)
  bram85/1 -> din_bussify/86(in86)
  bram86/1 -> din_bussify/87(in87)
  bram87/1 -> din_bussify/88(in88)
  bram88/1 -> din_bussify/89(in89)
  bram89/1 -> din_bussify/90(in90)
  bram90/1 -> din_bussify/91(in91)
  bram91/1 -> din_bussify/92(in92)
  bram92/1 -> din_bussify/93(in93)
  bram93/1 -> din_bussify/94(in94)
  bram94/1 -> din_bussify/95(in95)
  bram95/1 -> din_bussify/96(in96)
  bram96/1 -> din_bussify/97(in97)
  bram97/1 -> din_bussify/98(in98)
  bram98/1 -> din_bussify/99(in99)
  bram99/1 -> din_bussify/100(in100)
  bram100/1 -> din_bussify/101(in101)
  bram101/1 -> din_bussify/102(in102)
  bram102/1 -> din_bussify/103(in103)
  bram103/1 -> din_bussify/104(in104)
  bram104/1 -> din_bussify/105(in105)
  bram105/1 -> din_bussify/106(in106)
  bram106/1 -> din_bussify/107(in107)
  bram107/1 -> din_bussify/108(in108)
  bram108/1 -> din_bussify/109(in109)
  bram109/1 -> din_bussify/110(in110)
  bram110/1 -> din_bussify/111(in111)
  bram111/1 -> din_bussify/112(in112)
  bram112/1 -> din_bussify/113(in113)
  bram113/1 -> din_bussify/114(in114)
  bram114/1 -> din_bussify/115(in115)
  bram115/1 -> din_bussify/116(in116)
  bram116/1 -> din_bussify/117(in117)
  bram117/1 -> din_bussify/118(in118)
  bram118/1 -> din_bussify/119(in119)
  bram119/1 -> din_bussify/120(in120)
  bram120/1 -> din_bussify/121(in121)
  bram121/1 -> din_bussify/122(in122)
  bram122/1 -> din_bussify/123(in123)
  bram123/1 -> din_bussify/124(in124)
  bram124/1 -> din_bussify/125(in125)
  bram125/1 -> din_bussify/126(in126)
  din_bussify/1(bus_out) -> dout/1
  den/1 -> dvalid/1

== system snb_bc/pfb_fft/pfb_fir_generic/pfb_fir_taps/en_expand ==
  bus_in : Inport
  slice1 : xbsIndex_r4/Slice  nbits=1  boolean_output=on  mode=Upper Bit Location + Width  bit1=-1  base1=MSB of Input  bit0=0  base0=LSB of Input  dbl_ovrd=off  block_type=slice
  slice2 : xbsIndex_r4/Slice  nbits=1  boolean_output=on  mode=Upper Bit Location + Width  bit1=0  base1=MSB of Input  bit0=0  base0=LSB of Input  dbl_ovrd=off  block_type=slice
  msb_out2 : Outport
  lsb_out1 : Outport  Port=2
  wires:
  bus_in/1 -> slice2/1, slice1/1
  slice2/1 -> msb_out2/1
  slice1/1 -> lsb_out1/1

== system snb_bc/pfb_fft/pfb_fir_generic/pfb_fir_taps/en_replicate0 ==
  in : Inport
  bussify : Subsystem  AncestorBlock=casper_library_flow_control/bus_create  mask(bus_create){inputNum=14}
      mask prompts: inputNum "Number of inputs:"
      mask init:
      | bus_create_init(gcb,...
      |     'inputNum', inputNum);
  din0_0 : xbsIndex_r4/Delay  rst=off  infoeditControl=Selection of Reset will increase slice count due to use of real FFs and instead of SRLs  en=off  latency=1  dbl_ovrd=off  reg_retiming=off  block_type=delay
  din1_0 : xbsIndex_r4/Delay  rst=off  infoeditControl=Selection of Reset will increase slice count due to use of real FFs and instead of SRLs  en=off  latency=1  dbl_ovrd=off  reg_retiming=off  block_type=delay
  din1_1 : xbsIndex_r4/Delay  rst=off  infoeditControl=Selection of Reset will increase slice count due to use of real FFs and instead of SRLs  en=off  latency=1  dbl_ovrd=off  reg_retiming=off  block_type=delay
  din2_{0..3} (4 alike) : xbsIndex_r4/Delay  rst=off  infoeditControl=Selection of Reset will increase slice count due to use of real FFs and instead of SRLs  en=off  latency=1  dbl_ovrd=off  reg_retiming=off  block_type=delay
  din3_{0..7} (8 alike) : xbsIndex_r4/Delay  rst=off  infoeditControl=Selection of Reset will increase slice count due to use of real FFs and instead of SRLs  en=off  latency=1  dbl_ovrd=off  reg_retiming=off  block_type=delay
  din4_{0..13} (14 alike) : xbsIndex_r4/Delay  rst=off  infoeditControl=Selection of Reset will increase slice count due to use of real FFs and instead of SRLs  en=off  latency=1  dbl_ovrd=off  reg_retiming=on  block_type=delay
  din5_{0..13} (14 alike) : xbsIndex_r4/Delay  rst=off  infoeditControl=Selection of Reset will increase slice count due to use of real FFs and instead of SRLs  en=off  latency=1  dbl_ovrd=off  reg_retiming=on  block_type=delay
  din6_{0..13} (14 alike) : xbsIndex_r4/Delay  rst=off  infoeditControl=Selection of Reset will increase slice count due to use of real FFs and instead of SRLs  en=off  latency=1  dbl_ovrd=off  reg_retiming=on  block_type=delay
  din7_{0..13} (14 alike) : xbsIndex_r4/Delay  rst=off  infoeditControl=Selection of Reset will increase slice count due to use of real FFs and instead of SRLs  en=off  latency=1  dbl_ovrd=off  reg_retiming=on  block_type=delay
  din8_{0..13} (14 alike) : xbsIndex_r4/Delay  rst=off  infoeditControl=Selection of Reset will increase slice count due to use of real FFs and instead of SRLs  en=off  latency=1  dbl_ovrd=off  reg_retiming=off  block_type=delay
  out : Outport
  wires:
  bussify/1(bus_out) -> out/1
  din8_13/1 -> bussify/14(in14)
  din8_12/1 -> bussify/13(in13)
  din8_11/1 -> bussify/12(in12)
  din8_10/1 -> bussify/11(in11)
  din8_9/1 -> bussify/10(in10)
  din8_8/1 -> bussify/9(in9)
  din8_7/1 -> bussify/8(in8)
  din8_6/1 -> bussify/7(in7)
  din8_5/1 -> bussify/6(in6)
  din8_4/1 -> bussify/5(in5)
  din8_3/1 -> bussify/4(in4)
  din8_2/1 -> bussify/3(in3)
  din8_1/1 -> bussify/2(in2)
  din8_0/1 -> bussify/1(in1)
  din7_13/1 -> din8_13/1
  din7_12/1 -> din8_12/1
  din7_11/1 -> din8_11/1
  din7_10/1 -> din8_10/1
  din7_9/1 -> din8_9/1
  din7_8/1 -> din8_8/1
  din7_7/1 -> din8_7/1
  din7_6/1 -> din8_6/1
  din7_5/1 -> din8_5/1
  din7_4/1 -> din8_4/1
  din7_3/1 -> din8_3/1
  din7_2/1 -> din8_2/1
  din7_1/1 -> din8_1/1
  din7_0/1 -> din8_0/1
  din6_13/1 -> din7_13/1
  din6_12/1 -> din7_12/1
  din6_11/1 -> din7_11/1
  din6_10/1 -> din7_10/1
  din6_9/1 -> din7_9/1
  din6_8/1 -> din7_8/1
  din6_7/1 -> din7_7/1
  din6_6/1 -> din7_6/1
  din6_5/1 -> din7_5/1
  din6_4/1 -> din7_4/1
  din6_3/1 -> din7_3/1
  din6_2/1 -> din7_2/1
  din6_1/1 -> din7_1/1
  din6_0/1 -> din7_0/1
  din5_13/1 -> din6_13/1
  din5_12/1 -> din6_12/1
  din5_11/1 -> din6_11/1
  din5_10/1 -> din6_10/1
  din5_9/1 -> din6_9/1
  din5_8/1 -> din6_8/1
  din5_7/1 -> din6_7/1
  din5_6/1 -> din6_6/1
  din5_5/1 -> din6_5/1
  din5_4/1 -> din6_4/1
  din5_3/1 -> din6_3/1
  din5_2/1 -> din6_2/1
  din5_1/1 -> din6_1/1
  din5_0/1 -> din6_0/1
  din4_13/1 -> din5_13/1
  din4_12/1 -> din5_12/1
  din4_11/1 -> din5_11/1
  din4_10/1 -> din5_10/1
  din4_9/1 -> din5_9/1
  din4_8/1 -> din5_8/1
  din4_7/1 -> din5_7/1
  din4_6/1 -> din5_6/1
  din4_5/1 -> din5_5/1
  din4_4/1 -> din5_4/1
  din4_3/1 -> din5_3/1
  din4_2/1 -> din5_2/1
  din4_1/1 -> din5_1/1
  din4_0/1 -> din5_0/1
  din3_7/1 -> din4_7/1
  din3_6/1 -> din4_6/1
  din3_5/1 -> din4_13/1, din4_5/1
  din3_4/1 -> din4_12/1, din4_4/1
  din3_3/1 -> din4_11/1, din4_3/1
  din3_2/1 -> din4_10/1, din4_2/1
  din3_1/1 -> din4_9/1, din4_1/1
  din3_0/1 -> din4_8/1, din4_0/1
  din2_3/1 -> din3_7/1, din3_3/1
  din2_2/1 -> din3_6/1, din3_2/1
  din2_1/1 -> din3_5/1, din3_1/1
  din2_0/1 -> din3_4/1, din3_0/1
  din1_1/1 -> din2_3/1, din2_1/1
  din1_0/1 -> din2_2/1, din2_0/1
  din0_0/1 -> din1_1/1, din1_0/1
  in/1 -> din0_0/1

== system snb_bc/pfb_fft/pfb_fir_generic/pfb_fir_taps/en_replicate1 ==
  in : Inport
  bussify : Subsystem  AncestorBlock=casper_library_flow_control/bus_create  mask(bus_create){inputNum=16}
      mask prompts: inputNum "Number of inputs:"
      mask init:
      | bus_create_init(gcb,...
      |     'inputNum', inputNum);
  din0_0 : xbsIndex_r4/Delay  rst=off  infoeditControl=Selection of Reset will increase slice count due to use of real FFs and instead of SRLs  en=off  latency=1  dbl_ovrd=off  reg_retiming=off  block_type=delay
  din1_0 : xbsIndex_r4/Delay  rst=off  infoeditControl=Selection of Reset will increase slice count due to use of real FFs and instead of SRLs  en=off  latency=1  dbl_ovrd=off  reg_retiming=off  block_type=delay
  din1_1 : xbsIndex_r4/Delay  rst=off  infoeditControl=Selection of Reset will increase slice count due to use of real FFs and instead of SRLs  en=off  latency=1  dbl_ovrd=off  reg_retiming=off  block_type=delay
  din2_{0..3} (4 alike) : xbsIndex_r4/Delay  rst=off  infoeditControl=Selection of Reset will increase slice count due to use of real FFs and instead of SRLs  en=off  latency=1  dbl_ovrd=off  reg_retiming=off  block_type=delay
  din3_{0..7} (8 alike) : xbsIndex_r4/Delay  rst=off  infoeditControl=Selection of Reset will increase slice count due to use of real FFs and instead of SRLs  en=off  latency=1  dbl_ovrd=off  reg_retiming=off  block_type=delay
  din4_{0..15} (16 alike) : xbsIndex_r4/Delay  rst=off  infoeditControl=Selection of Reset will increase slice count due to use of real FFs and instead of SRLs  en=off  latency=1  dbl_ovrd=off  reg_retiming=on  block_type=delay
  din5_{0..15} (16 alike) : xbsIndex_r4/Delay  rst=off  infoeditControl=Selection of Reset will increase slice count due to use of real FFs and instead of SRLs  en=off  latency=1  dbl_ovrd=off  reg_retiming=on  block_type=delay
  din6_{0..15} (16 alike) : xbsIndex_r4/Delay  rst=off  infoeditControl=Selection of Reset will increase slice count due to use of real FFs and instead of SRLs  en=off  latency=1  dbl_ovrd=off  reg_retiming=on  block_type=delay
  din7_{0..15} (16 alike) : xbsIndex_r4/Delay  rst=off  infoeditControl=Selection of Reset will increase slice count due to use of real FFs and instead of SRLs  en=off  latency=1  dbl_ovrd=off  reg_retiming=on  block_type=delay
  din8_{0..15} (16 alike) : xbsIndex_r4/Delay  rst=off  infoeditControl=Selection of Reset will increase slice count due to use of real FFs and instead of SRLs  en=off  latency=1  dbl_ovrd=off  reg_retiming=off  block_type=delay
  out : Outport
  wires:
  bussify/1(bus_out) -> out/1
  din8_15/1 -> bussify/16(in16)
  din8_14/1 -> bussify/15(in15)
  din8_13/1 -> bussify/14(in14)
  din8_12/1 -> bussify/13(in13)
  din8_11/1 -> bussify/12(in12)
  din8_10/1 -> bussify/11(in11)
  din8_9/1 -> bussify/10(in10)
  din8_8/1 -> bussify/9(in9)
  din8_7/1 -> bussify/8(in8)
  din8_6/1 -> bussify/7(in7)
  din8_5/1 -> bussify/6(in6)
  din8_4/1 -> bussify/5(in5)
  din8_3/1 -> bussify/4(in4)
  din8_2/1 -> bussify/3(in3)
  din8_1/1 -> bussify/2(in2)
  din8_0/1 -> bussify/1(in1)
  din7_15/1 -> din8_15/1
  din7_14/1 -> din8_14/1
  din7_13/1 -> din8_13/1
  din7_12/1 -> din8_12/1
  din7_11/1 -> din8_11/1
  din7_10/1 -> din8_10/1
  din7_9/1 -> din8_9/1
  din7_8/1 -> din8_8/1
  din7_7/1 -> din8_7/1
  din7_6/1 -> din8_6/1
  din7_5/1 -> din8_5/1
  din7_4/1 -> din8_4/1
  din7_3/1 -> din8_3/1
  din7_2/1 -> din8_2/1
  din7_1/1 -> din8_1/1
  din7_0/1 -> din8_0/1
  din6_15/1 -> din7_15/1
  din6_14/1 -> din7_14/1
  din6_13/1 -> din7_13/1
  din6_12/1 -> din7_12/1
  din6_11/1 -> din7_11/1
  din6_10/1 -> din7_10/1
  din6_9/1 -> din7_9/1
  din6_8/1 -> din7_8/1
  din6_7/1 -> din7_7/1
  din6_6/1 -> din7_6/1
  din6_5/1 -> din7_5/1
  din6_4/1 -> din7_4/1
  din6_3/1 -> din7_3/1
  din6_2/1 -> din7_2/1
  din6_1/1 -> din7_1/1
  din6_0/1 -> din7_0/1
  din5_15/1 -> din6_15/1
  din5_14/1 -> din6_14/1
  din5_13/1 -> din6_13/1
  din5_12/1 -> din6_12/1
  din5_11/1 -> din6_11/1
  din5_10/1 -> din6_10/1
  din5_9/1 -> din6_9/1
  din5_8/1 -> din6_8/1
  din5_7/1 -> din6_7/1
  din5_6/1 -> din6_6/1
  din5_5/1 -> din6_5/1
  din5_4/1 -> din6_4/1
  din5_3/1 -> din6_3/1
  din5_2/1 -> din6_2/1
  din5_1/1 -> din6_1/1
  din5_0/1 -> din6_0/1
  din4_15/1 -> din5_15/1
  din4_14/1 -> din5_14/1
  din4_13/1 -> din5_13/1
  din4_12/1 -> din5_12/1
  din4_11/1 -> din5_11/1
  din4_10/1 -> din5_10/1
  din4_9/1 -> din5_9/1
  din4_8/1 -> din5_8/1
  din4_7/1 -> din5_7/1
  din4_6/1 -> din5_6/1
  din4_5/1 -> din5_5/1
  din4_4/1 -> din5_4/1
  din4_3/1 -> din5_3/1
  din4_2/1 -> din5_2/1
  din4_1/1 -> din5_1/1
  din4_0/1 -> din5_0/1
  din3_7/1 -> din4_15/1, din4_7/1
  din3_6/1 -> din4_14/1, din4_6/1
  din3_5/1 -> din4_13/1, din4_5/1
  din3_4/1 -> din4_12/1, din4_4/1
  din3_3/1 -> din4_11/1, din4_3/1
  din3_2/1 -> din4_10/1, din4_2/1
  din3_1/1 -> din4_9/1, din4_1/1
  din3_0/1 -> din4_8/1, din4_0/1
  din2_3/1 -> din3_7/1, din3_3/1
  din2_2/1 -> din3_6/1, din3_2/1
  din2_1/1 -> din3_5/1, din3_1/1
  din2_0/1 -> din3_4/1, din3_0/1
  din1_1/1 -> din2_3/1, din2_1/1
  din1_0/1 -> din2_2/1, din2_0/1
  din0_0/1 -> din1_1/1, din1_0/1
  in/1 -> din0_0/1
